simulink subsystem "CrazyfliePlant"  (R2024a)
settings: Solver=VariableStepAuto  StartTime=0.0  StopTime=10.0  RelTol=1e-3
undefined symbols (not defined in the file): d, g, I, k_q, k_t, m, rad, s
libraries: aerolibutil x5, aerolibconvert2 x4, matrix_library x1, sharedutil x1
settings Model: Creator=dylanfanner  LastModifiedBy=User

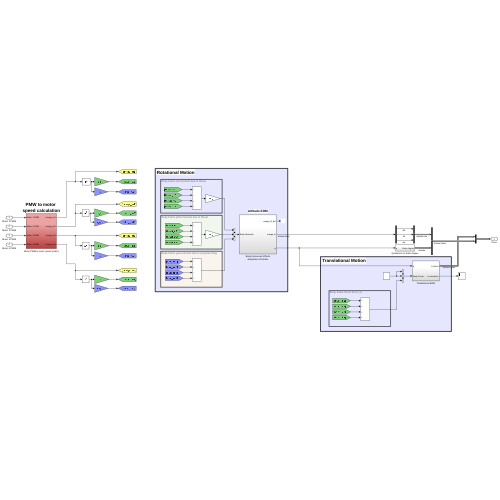
[thumbnail: Simulink's stored preview of the top-level diagram]
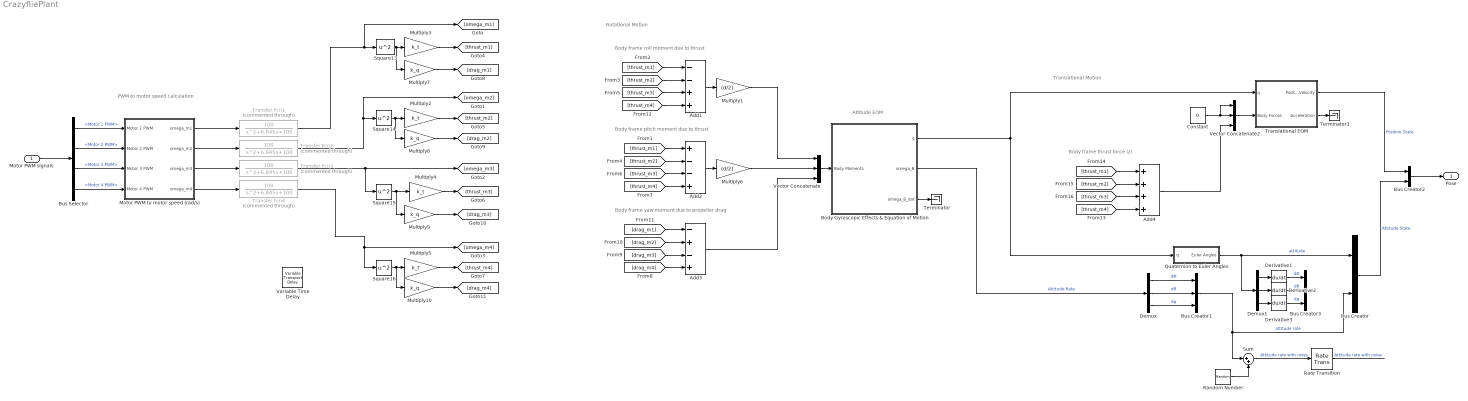
== system CrazyfliePlant ==
  note: Body frame pitch moment due to thrust
  note: Translational Motion
  note: Body frame thrust force (z)
  note: Body frame roll moment due to thrust
  note: Body frame yaw moment due to propeller drag
  note: PWM to motor
      | speed calculation
  note: Rotational Motion
  note: Attitude EOM
  Motor PWM signals : Inport
  Add1 : Sum  Inputs=--++
  Add2 : Sum  Inputs=+--+
  Add3 : Sum  Inputs=-+-+
  Add4 : Sum  Inputs=++++
  Body Gyroscopic Effects & Equation of Motion : Subsystem
  Bus Creator : BusCreator  Inputs=2
  Bus Creator1 : BusCreator  Inputs=3
  Bus Creator2 : BusCreator  Inputs=2
  Bus Creator3 : BusCreator  Inputs=3
  Bus Selector : BusSelector  OutputSignals=Motor 1 PWM,Motor 2 PWM,Motor 3 PWM,Motor 4 PWM
  Constant : Constant  Value=0
  Demux : Demux  Outputs=3
  Demux1 : Demux  Outputs=3
  Derivative1 : Derivative
  Derivative2 : Derivative
  Derivative3 : Derivative
  Motor PWM to motor speed (rad/s) : Subsystem
  Multiply1 : Gain  Gain=(d/2)
  Multiply{7..10} (4 alike) : Gain  Gain=k_q
  Multiply{2..5} (4 alike) : Gain  Gain=k_t
  Multiply6 : Gain  Gain=(d/2)
  Quaternion to Euler Angles : Subsystem
  Random Number : RandomNumber  Variance=0.00005  SampleTime=0.001
  Rate Transition : RateTransition  OutPortSampleTime=0.01
  Square{13..16} (4 alike) : Math  Operator=square
  Sum : Sum  Inputs=|++
  Terminator : Terminator
  Terminator1 : Terminator
  Transfer Fcn{1..4} (4 alike) : TransferFcn  Commented=through  Numerator=100  Denominator=[1 6.845 100]
  Translational EOM : Subsystem
  Variable Time Delay : VariableTransportDelay  MaximumDelay=10
  Vector Concatenate : Concatenate  NumInputs=3
  Vector Concatenate2 : Concatenate  NumInputs=3
  Pose : Outport
  wires:
  Constant/1 -> Vector Concatenate2/1, Vector Concatenate2/2
  Demux/2 -> Bus Creator1/2  "dθ"
  Multiply8/1 -> [drag_m2]
  [thrust_m3] -> Add1/3
  [thrust_m2] -> Add2/2
  Vector Concatenate/1 -> Body Gyroscopic Effects & Equation of Motion/1(Body Moments)
  [thrust_m3] -> Add4/3
  [thrust_m1] -> Add4/1
  [thrust_m1] -> Add1/1
  [thrust_m1] -> Add2/1
  [thrust_m4] -> Add2/4
  Multiply7/1 -> [drag_m1]
  Demux/1 -> Bus Creator1/1  "dΦ"
  Add2/1 -> Multiply6/1
  Bus Creator/1 -> Bus Creator2/2  "Attitude State"
  Square14/1 -> Multiply2/1, Multiply8/1
  [drag_m2] -> Add3/2
  Quaternion to Euler Angles/1(Euler Angles) -> Bus Creator/1, Demux1/1  "attitude"
  Square16/1 -> Multiply5/1, Multiply10/1
  Multiply4/1 -> [thrust_m3]
  Multiply2/1 -> [thrust_m2]
  [thrust_m4] -> Add1/4
  Body Gyroscopic Effects & Equation of Motion/1(q) -> Translational EOM/1(q), Quaternion to Euler Angles/1(q)
  Add4/1 -> Vector Concatenate2/3
  Translational EOM/2(Acceleration) -> Terminator1/1
  Multiply10/1 -> [drag_m4]
  [thrust_m4] -> Add4/4
  [thrust_m2] -> Add4/2
  Multiply5/1 -> [thrust_m4]
  [drag_m3] -> Add3/3
  Multiply9/1 -> [drag_m3]
  [thrust_m2] -> Add1/2
  Body Gyroscopic Effects & Equation of Motion/2(omega_B) -> Demux/1  "Attitude Rate"
  Square15/1 -> Multiply4/1, Multiply9/1
  Body Gyroscopic Effects & Equation of Motion/3(omega_B_dot) -> Terminator/1
  Translational EOM/1(Position&Velocity) -> Bus Creator2/1  "Position State"
  Bus Creator1/1 -> Bus Creator/2, Sum/1  "attitude rate"
  [drag_m1] -> Add3/1
  [thrust_m3] -> Add2/3
  Vector Concatenate2/1 -> Translational EOM/2(Body Forces)
  Bus Creator2/1 -> Pose/1
  Multiply3/1 -> [thrust_m1]
  Square13/1 -> Multiply7/1, Multiply3/1
  Add1/1 -> Multiply1/1
  [drag_m4] -> Add3/4
  Motor PWM signals/1 -> Bus Selector/1
  Bus Selector/4 -> Motor PWM to motor speed (rad/s)/4(Motor 4 PWM)  "<Motor 4 PWM>"
  Bus Selector/3 -> Motor PWM to motor speed (rad/s)/3(Motor 3 PWM)  "<Motor 3 PWM>"
  Bus Selector/2 -> Motor PWM to motor speed (rad/s)/2(Motor 2 PWM)  "<Motor 2 PWM>"
  Bus Selector/1 -> Motor PWM to motor speed (rad/s)/1(Motor 1 PWM)  "<Motor 1 PWM>"
  Demux/3 -> Bus Creator1/3  "dψ"
  Random Number/1 -> Sum/2
  Sum/1 -> Rate Transition/1  "Attitude rate with noise"
  Rate Transition/1 -> ?  "Attitude rate with noise"
  Motor PWM to motor speed (rad/s)/2(omega_m2) -> Transfer Fcn2/1
  Motor PWM to motor speed (rad/s)/1(omega_m1) -> Transfer Fcn1/1
  Motor PWM to motor speed (rad/s)/4(omega_m4) -> Transfer Fcn4/1
  Motor PWM to motor speed (rad/s)/3(omega_m3) -> Transfer Fcn3/1
  Transfer Fcn1/1 -> Square13/1, [omega_m1]
  Transfer Fcn2/1 -> Square14/1, [omega_m2]
  Transfer Fcn3/1 -> Square15/1, [omega_m3]
  Transfer Fcn4/1 -> Square16/1, [omega_m4]
  Multiply1/1 -> Vector Concatenate/1
  Multiply6/1 -> Vector Concatenate/2
  Add3/1 -> Vector Concatenate/3
  Demux1/3 -> Derivative3/1
  Demux1/1 -> Derivative1/1
  Demux1/2 -> Derivative2/1
  Derivative1/1 -> Bus Creator3/1  "dΦ"
  Derivative2/1 -> Bus Creator3/2  "dθ"
  Derivative3/1 -> Bus Creator3/3  "dψ"

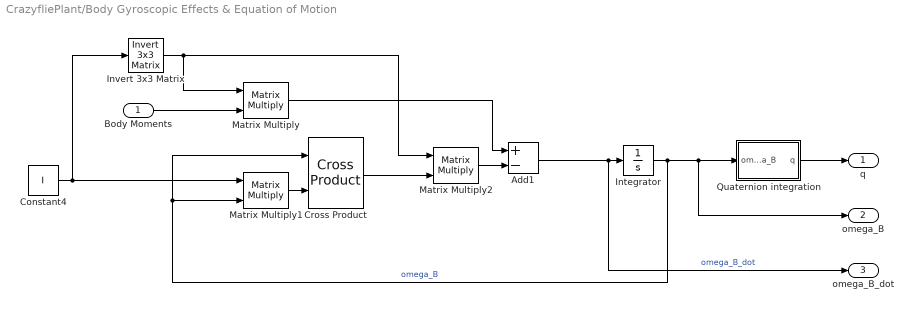
== system CrazyfliePlant/Body Gyroscopic Effects & Equation of Motion ==
  Body Moments : Inport
  Add1 : Sum  Inputs=+-
  Constant4 : Constant  Value=I
  Cross Product : matrix_library/Cross Product
  Integrator : Integrator
  Invert 3x3 Matrix : aerolibutil/Invert  3x3 Matrix
  Matrix Multiply : Product  Multiplication=Matrix(*)
  Matrix Multiply1 : Product  Multiplication=Matrix(*)
  Matrix Multiply2 : Product  Multiplication=Matrix(*)
  Quaternion integration : Subsystem
  q : Outport
  omega_B : Outport  Port=2
  omega_B_dot : Outport  Port=3
  wires:
  Constant4/1 -> Invert 3x3 Matrix/1, Matrix Multiply1/1
  Add1/1 -> Integrator/1, omega_B_dot/1  "omega_B_dot"
  Matrix Multiply2/1 -> Add1/2
  Matrix Multiply1/1 -> Cross Product/2
  Matrix Multiply/1 -> Add1/1
  Cross Product/1 -> Matrix Multiply2/2
  Integrator/1 -> omega_B/1, Quaternion integration/1(omega_B), Cross Product/1, Matrix Multiply1/2  "omega_B"
  Invert 3x3 Matrix/1 -> Matrix Multiply2/1, Matrix Multiply/1
  Body Moments/1 -> Matrix Multiply/2
  Quaternion integration/1(q) -> q/1

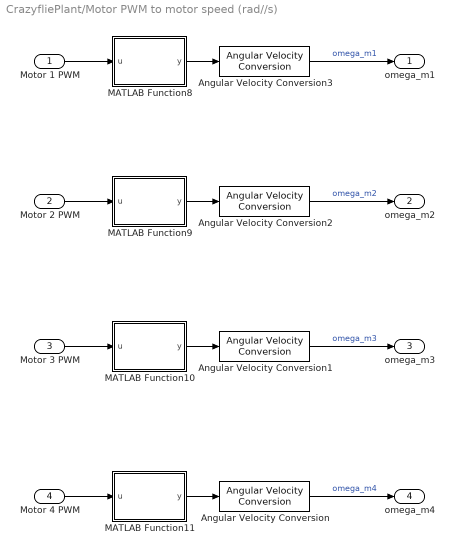
== system CrazyfliePlant/Motor PWM to motor speed (rad//s) ==
  Motor 1 PWM : Inport
  Motor 2 PWM : Inport  Port=2
  Motor 3 PWM : Inport  Port=3
  Motor 4 PWM : Inport  Port=4
  Angular Velocity Conversion{,1..3} (4 alike) : aerolibconvert2/Angular Velocity Conversion  IU=rpm  OU=rad/s
  MATLAB Function10 : MATLAB Function  TreatAsAtomicUnit=on
  MATLAB Function11 : MATLAB Function  TreatAsAtomicUnit=on
  MATLAB Function8 : MATLAB Function  TreatAsAtomicUnit=on
  MATLAB Function9 : MATLAB Function  TreatAsAtomicUnit=on
  omega_m1 : Outport
  omega_m2 : Outport  Port=2
  omega_m3 : Outport  Port=3
  omega_m4 : Outport  Port=4
  wires:
  MATLAB Function9/1(y) -> Angular Velocity Conversion2/1
  Angular Velocity Conversion1/1 -> omega_m3/1  "omega_m3"
  Angular Velocity Conversion/1 -> omega_m4/1  "omega_m4"
  MATLAB Function11/1(y) -> Angular Velocity Conversion/1
  Angular Velocity Conversion2/1 -> omega_m2/1  "omega_m2"
  MATLAB Function8/1(y) -> Angular Velocity Conversion3/1
  Angular Velocity Conversion3/1 -> omega_m1/1  "omega_m1"
  MATLAB Function10/1(y) -> Angular Velocity Conversion1/1
  Motor 1 PWM/1 -> MATLAB Function8/1(u)
  Motor 2 PWM/1 -> MATLAB Function9/1(u)
  Motor 3 PWM/1 -> MATLAB Function10/1(u)
  Motor 4 PWM/1 -> MATLAB Function11/1(u)

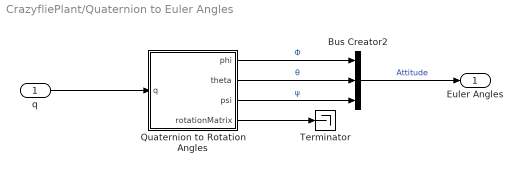
== system CrazyfliePlant/Quaternion to Euler Angles ==
  q : Inport
  Bus Creator2 : BusCreator  Inputs=3
  Quaternion to Rotation Angles : MATLAB Function  TreatAsAtomicUnit=on
  Terminator : Terminator
  Euler Angles : Outport
  wires:
  Bus Creator2/1 -> Euler Angles/1  "Attitude"
  Quaternion to Rotation Angles/1(phi) -> Bus Creator2/1  "Φ"
  Quaternion to Rotation Angles/3(psi) -> Bus Creator2/3  "ψ"
  Quaternion to Rotation Angles/2(theta) -> Bus Creator2/2  "θ"
  q/1 -> Quaternion to Rotation Angles/1(q)
  Quaternion to Rotation Angles/4(rotationMatrix) -> Terminator/1

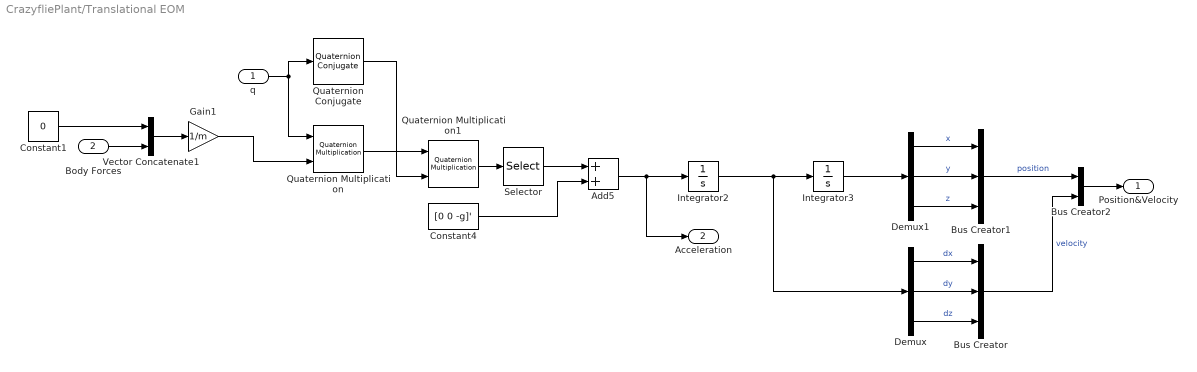
== system CrazyfliePlant/Translational EOM ==
  q : Inport
  Body Forces : Inport  Port=2
  Add5 : Sum
  Bus Creator : BusCreator  Inputs=3
  Bus Creator1 : BusCreator  Inputs=3
  Bus Creator2 : BusCreator  Inputs=2
  Constant1 : Constant  Value=0
  Constant4 : Constant  Value=[0 0 -g]'
  Demux : Demux  Outputs=3
  Demux1 : Demux  Outputs=3
  Gain1 : Gain  Gain=1/m
  Integrator2 : Integrator
  Integrator3 : Integrator  InitialCondition=[0 0 0]
  Quaternion Conjugate : aerolibutil/Quaternion Conjugate
  Quaternion Multiplication : aerolibutil/Quaternion Multiplication
  Quaternion Multiplication1 : aerolibutil/Quaternion Multiplication
  Selector : Selector  InputPortWidth=4  IndexOptions=Index vector (dialog)  Indices=[2 3 4]  OutputSizes=1
  Vector Concatenate1 : Concatenate
  Position&Velocity : Outport
  Acceleration : Outport  Port=2
  wires:
  Bus Creator/1 -> Bus Creator2/2  "velocity"
  Gain1/1 -> Quaternion Multiplication/2
  Constant1/1 -> Vector Concatenate1/1
  Quaternion Conjugate/1 -> Quaternion Multiplication1/2
  Selector/1 -> Add5/1
  Quaternion Multiplication/1 -> Quaternion Multiplication1/1
  q/1 -> Quaternion Multiplication/1, Quaternion Conjugate/1
  Quaternion Multiplication1/1 -> Selector/1
  Vector Concatenate1/1 -> Gain1/1
  Body Forces/1 -> Vector Concatenate1/2
  Add5/1 -> Integrator2/1, Acceleration/1
  Demux/1 -> Bus Creator/1  "dx"
  Demux/2 -> Bus Creator/2  "dy"
  Demux/3 -> Bus Creator/3  "dz"
  Bus Creator1/1 -> Bus Creator2/1  "position"
  Demux1/1 -> Bus Creator1/1  "x"
  Demux1/2 -> Bus Creator1/2  "y"
  Demux1/3 -> Bus Creator1/3  "z"
  Bus Creator2/1 -> Position&Velocity/1
  Integrator2/1 -> Demux/1, Integrator3/1
  Integrator3/1 -> Demux1/1
  Constant4/1 -> Add5/2

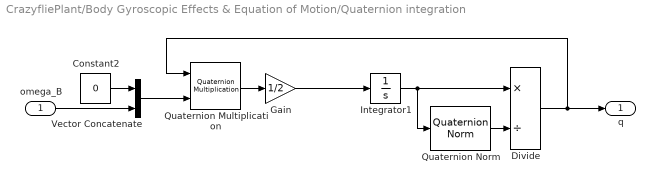
== system CrazyfliePlant/Body Gyroscopic Effects & Equation of Motion/Quaternion integration ==
  omega_B : Inport
  Constant2 : Constant  Value=0
  Divide : Product  Inputs=*/
  Gain : Gain  Gain=1/2
  Integrator1 : Integrator  InitialCondition=[1 0 0 0]'
  Quaternion Multiplication : aerolibutil/Quaternion Multiplication
  Quaternion Norm : sharedutil/Quaternion Norm  aMode=aMode
      settings: LibrarySourceBlock=|
      | aerolibutil/Quaternion
      | Norm
  Vector Concatenate : Concatenate
  q : Outport
  wires:
  Divide/1 -> Quaternion Multiplication/1, q/1
  Integrator1/1 -> Quaternion Norm/1, Divide/1
  Constant2/1 -> Vector Concatenate/1
  Quaternion Multiplication/1 -> Gain/1
  Vector Concatenate/1 -> Quaternion Multiplication/2
  Gain/1 -> Integrator1/1
  Quaternion Norm/1 -> Divide/2
  omega_B/1 -> Vector Concatenate/2

== matlab function CrazyfliePlant/Motor PWM to motor speed (rad//s)/MATLAB Function10 ==
  data: u input; y output
function y = PWMtoRPM(u)

y = u*0.2685+4070.3;

== matlab function CrazyfliePlant/Motor PWM to motor speed (rad//s)/MATLAB Function11 ==
  data: u input; y output
function y = PWMtoRPM(u)

y = u*0.2685+4070.3;

== matlab function CrazyfliePlant/Motor PWM to motor speed (rad//s)/MATLAB Function8 ==
  data: u input; y output
function y = PWMtoRPM(u)

y = u*0.2685+4070.3;

== matlab function CrazyfliePlant/Motor PWM to motor speed (rad//s)/MATLAB Function9 ==
  data: u input; y output
function y = PWMtoRPM(u)

y = u*0.2685+4070.3;

== matlab function CrazyfliePlant/Quaternion to Euler Angles/Quaternion to Rotation Angles ==
  data: q input; phi output; theta output; psi output; rotationMatrix output
function [phi, theta, psi, rotationMatrix] = fcn(q)

q_0 = q(1);
q_x = q(2);
q_y = q(3);
q_z = q(4);

R_11 = 2*(q_0^2 + q_x^2) - 1;
R_12 = 2*(q_x*q_y - q_0*q_z);
R_13 = 2*(q_x*q_z + q_0*q_y);

R_21 = 2*(q_x*q_y + q_0*q_z);
R_22 = 2*(q_0^2 + q_y^2) - 1;
R_23 = 2*(q_y*q_z - q_0*q_x);

R_31 = 2*(q_x*q_z - q_0*q_y);
R_32 = 2*(q_y*q_z + q_0*q_x);
R_33 = 2*(q_0^2 + q_z^2) - 1;

phi = atan2(R_32, R_33);
theta = -atan2(R_31, sqrt(1 - (R_31^2)));
psi = atan2(R_21, R_11);

rotationMatrix = [R_11 R_12 R_13;...
        R_21 R_22 R_23;...
        R_31 R_32 R_33];
